simulink model "ZynqBF_2tx_fpga"  (R2018b)
settings: Solver=FixedStepDiscrete  StartTime=0.0  StopTime=10.0  FixedStep=(1/420e3)/128  RelTol=1e-3
undefined symbols (not defined in the file): a, b, c, gs1_i, gs1_q, gs2_i, gs2_q, gs_length
libraries: hdlsllib x65, simulink x41
(part 1 of 4)
settings Model: DataTypeOverride=Off  Creator=jason  LastModifiedBy=meyer
settings DataIOCC: SaveOutput=off  SaveTime=off
settings OptimizationCC: BlockReduction=off  ConditionallyExecuteInputs=off  DefaultParameterBehavior=Inlined
settings DebuggingCC: AlgebraicLoopMsg=error  SingleTaskRateTransMsg=error  ParameterPrecisionLossMsg=none  StrictBusMsg=ErrorOnBusTreatedAsVector
settings HardwareCC: ProdBitPerPointer=32  ProdBitPerSizeT=32  ProdBitPerPtrDiffT=32  ProdLargestAtomicFloat=None  ProdIntDivRoundTo=Undefined  ProdEndianess=Unspecified  ProdWordSize=32  ProdHWDeviceType=ASIC/FPGA->ASIC/FPGA  ProdEqTarget=off
settings SFSimCC: SimUseLocalCustomCode=off
settings RTWCC: RTWUseLocalCustomCode=off
settings CodeAppCC: StateflowObjectComments=on
settings GRTTargetCC: TargetLangStandard=C89/C90 (ANSI)

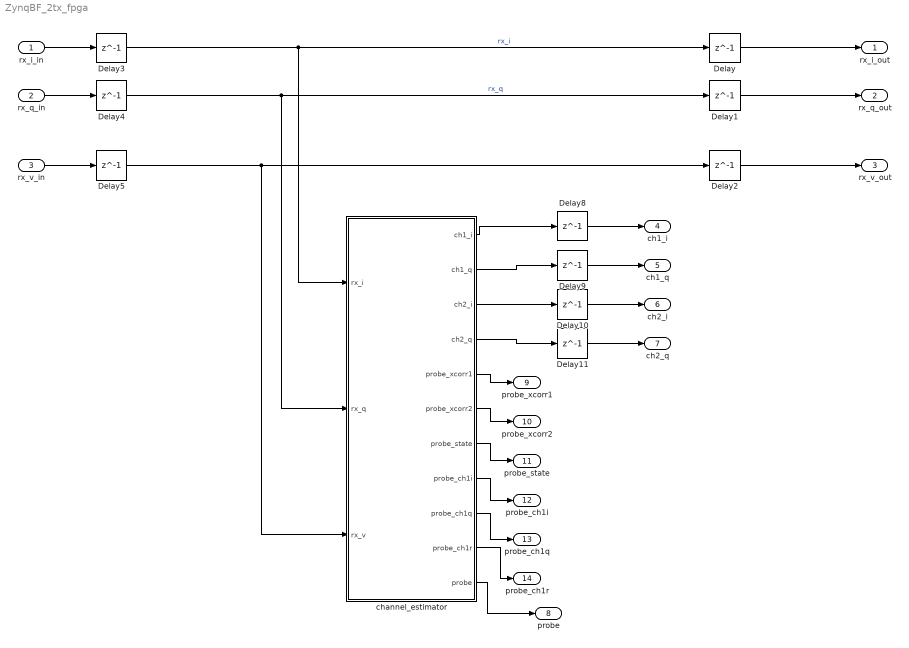
== system ZynqBF_2tx_fpga ==
  rx_i_in : Inport  OutDataTypeStr=fixdt(1,16,15)  SampleTime=1/420e3
  rx_q_in : Inport  Port=2  OutDataTypeStr=fixdt(1,16,15)  SampleTime=1/420e3
  rx_v_in : Inport  Port=3  OutDataTypeStr=boolean  SampleTime=1/420e3
  Delay{,1..5,8..11} (10 alike) : Delay  DelayLength=1
  channel_estimator : Subsystem  TreatAsAtomicUnit=on
  rx_i_out : Outport  OutDataTypeStr=fixdt(1,16,15)  SampleTime=1/420e3
  rx_q_out : Outport  Port=2  OutDataTypeStr=fixdt(1,16,15)  SampleTime=1/420e3
  rx_v_out : Outport  Port=3  OutDataTypeStr=boolean  SampleTime=1/420e3  LockScale=on
  ch1_i : Outport  Port=4  OutDataTypeStr=fixdt(1,16,15)
  ch1_q : Outport  Port=5  OutDataTypeStr=fixdt(1,16,15)
  ch2_i : Outport  Port=6  OutDataTypeStr=fixdt(1,16,15)
  ch2_q : Outport  Port=7  OutDataTypeStr=fixdt(1,16,15)
  probe : Outport  Port=8
  probe_xcorr1 : Outport  Port=9
  probe_xcorr2 : Outport  Port=10
  probe_state : Outport  Port=11
  probe_ch1i : Outport  Port=12
  probe_ch1q : Outport  Port=13
  probe_ch1r : Outport  Port=14
  wires:
  rx_i_in/1 -> Delay3/1
  rx_q_in/1 -> Delay4/1
  rx_v_in/1 -> Delay5/1
  Delay/1 -> rx_i_out/1
  Delay1/1 -> rx_q_out/1
  Delay2/1 -> rx_v_out/1
  channel_estimator/1(ch1_i) -> Delay8/1
  channel_estimator/2(ch1_q) -> Delay9/1
  channel_estimator/3(ch2_i) -> Delay10/1
  channel_estimator/4(ch2_q) -> Delay11/1
  Delay4/1 -> channel_estimator/2(rx_q), Delay1/1  "rx_q"
  Delay5/1 -> channel_estimator/3(rx_v), Delay2/1
  Delay8/1 -> ch1_i/1
  Delay9/1 -> ch1_q/1
  Delay10/1 -> ch2_i/1
  Delay11/1 -> ch2_q/1
  Delay3/1 -> channel_estimator/1(rx_i), Delay/1  "rx_i"
  channel_estimator/5(probe_xcorr1) -> probe_xcorr1/1
  channel_estimator/6(probe_xcorr2) -> probe_xcorr2/1
  channel_estimator/7(probe_state) -> probe_state/1
  channel_estimator/8(probe_ch1i) -> probe_ch1i/1
  channel_estimator/9(probe_ch1q) -> probe_ch1q/1
  channel_estimator/10(probe_ch1r) -> probe_ch1r/1
  channel_estimator/11(probe) -> probe/1

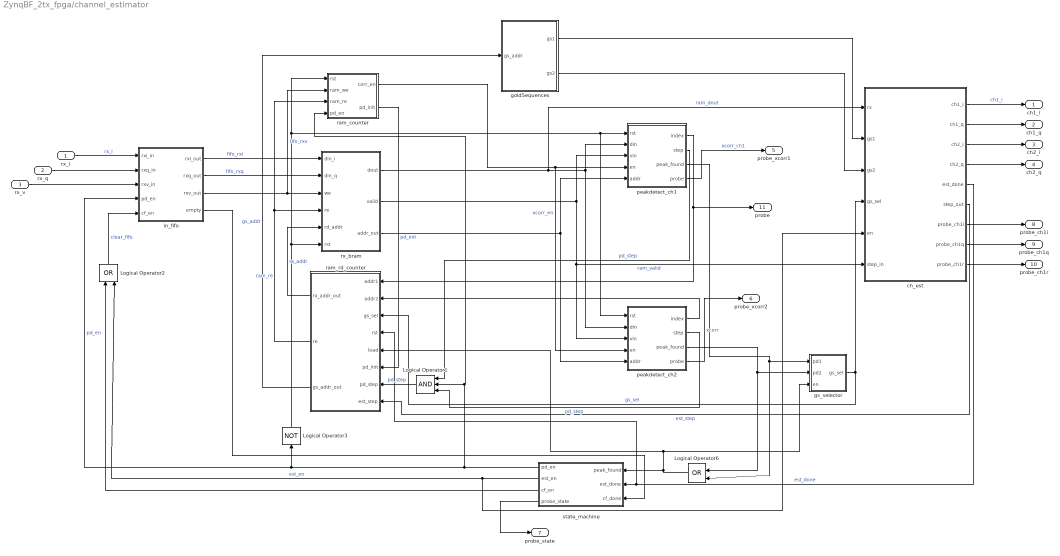
== system ZynqBF_2tx_fpga/channel_estimator ==
  rx_i : Inport
  rx_q : Inport  Port=2
  rx_v : Inport  Port=3
  Logical Operator1 : Logic  Inputs=3  IconShape=distinctive  AllPortsSameDT=off  OutDataTypeStr=boolean
  Logical Operator2 : Logic  Operator=OR  IconShape=distinctive  AllPortsSameDT=off  OutDataTypeStr=boolean
  Logical Operator3 : Logic  Operator=NOT  IconShape=distinctive  AllPortsSameDT=off  OutDataTypeStr=boolean
  Logical Operator6 : Logic  Operator=OR  IconShape=distinctive  AllPortsSameDT=off  OutDataTypeStr=boolean
  ch_est : Subsystem
  goldSequences : Subsystem
  gs_selector : Subsystem
  in_fifo : Subsystem
  peakdetect_ch1 : Subsystem
  peakdetect_ch2 : Subsystem
  ram_counter : Subsystem
  ram_rd_counter : Subsystem
  rx_bram : Subsystem
  state_machine : Subsystem
  ch1_i : Outport
  ch1_q : Outport  Port=2
  ch2_i : Outport  Port=3
  ch2_q : Outport  Port=4
  probe_xcorr1 : Outport  Port=5
  probe_xcorr2 : Outport  Port=6
  probe_state : Outport  Port=7
  probe_ch1i : Outport  Port=8
  probe_ch1q : Outport  Port=9
  probe_ch1r : Outport  Port=10
  probe : Outport  Port=11
  wires:
  in_fifo/3(rxv_out) -> ram_counter/2(ram_we), rx_bram/3(we)  "fifo_rxv"
  peakdetect_ch1/2(step) -> Logical Operator1/1  "pd_step"
  rx_bram/1(dout) -> ch_est/1(rx), peakdetect_ch2/2(din), peakdetect_ch1/2(din)  "ram_dout"
  goldSequences/1(gs1) -> ch_est/2(gs1)
  state_machine/1(pd_en) -> Logical Operator3/1, in_fifo/4(pd_en), ram_counter/4(pd_en), Logical Operator1/2  "pd_en"
  Logical Operator6/1 -> state_machine/1(peak_found), ram_rd_counter/5(load), gs_selector/3(en)
  ch_est/5(est_done) -> ram_rd_counter/4(rst), state_machine/2(est_done)  "est_done"
  goldSequences/2(gs2) -> ch_est/3(gs2)
  peakdetect_ch2/3(peak_found) -> Logical Operator6/1, gs_selector/2(pd2)
  peakdetect_ch1/3(peak_found) -> Logical Operator6/2, gs_selector/1(pd1)
  gs_selector/1(gs_sel) -> ch_est/4(gs_sel), ram_rd_counter/3(gs_sel)  "gs_sel"
  ch_est/1(ch1_i) -> ch1_i/1  "ch1_i"
  ch_est/2(ch1_q) -> ch1_q/1
  ch_est/3(ch2_i) -> ch2_i/1
  ch_est/4(ch2_q) -> ch2_q/1
  rx_bram/2(valid) -> peakdetect_ch2/3(vin), ch_est/6(step_in), peakdetect_ch1/3(vin)  "ram_valid"
  ram_rd_counter/1(rx_addr_out) -> rx_bram/5(rd_addr)  "rx_addr"
  ram_rd_counter/2(re) -> ram_counter/3(ram_re), rx_bram/4(re)  "ram_re"
  state_machine/2(est_en) -> ch_est/5(en), Logical Operator2/2  "est_en"
  rx_bram/3(addr_out) -> peakdetect_ch2/5(addr), peakdetect_ch1/5(addr)
  ram_rd_counter/3(gs_addr_out) -> goldSequences/1(gs_addr)  "gs_addr"
  ch_est/6(step_out) -> ram_rd_counter/8(est_step)  "est_step"
  peakdetect_ch2/2(step) -> Logical Operator1/3  "pd_step"
  peakdetect_ch1/1(index) -> probe/1, ram_rd_counter/1(addr1)
  peakdetect_ch2/1(index) -> ram_rd_counter/2(addr2)
  peakdetect_ch2/4(probe) -> probe_xcorr2/1  "xcorr"
  state_machine/3(cf_en) -> Logical Operator2/1
  peakdetect_ch1/4(probe) -> probe_xcorr1/1  "xcorr_ch1"
  ram_counter/1(corr_en) -> peakdetect_ch2/4(en), peakdetect_ch1/4(en)  "xcorr_en"
  in_fifo/1(rxi_out) -> rx_bram/1(din_i)  "fifo_rxi"
  in_fifo/2(rxq_out) -> rx_bram/2(din_q)  "fifo_rxq"
  rx_i/1 -> in_fifo/1(rxi_in)  "rx_i"
  rx_q/1 -> in_fifo/2(rxq_in)
  rx_v/1 -> in_fifo/3(rxv_in)
  in_fifo/4(empty) -> state_machine/3(cf_done)
  Logical Operator2/1 -> in_fifo/5(cf_en)  "clear_fifo"
  ch_est/7(probe_ch1i) -> probe_ch1i/1
  ch_est/8(probe_ch1q) -> probe_ch1q/1
  ch_est/9(probe_ch1r) -> probe_ch1r/1
  state_machine/4(probe_state) -> probe_state/1
  Logical Operator3/1 -> ram_counter/1(rst), peakdetect_ch2/1(rst), peakdetect_ch1/1(rst), rx_bram/6(rst)
  ram_counter/2(pd_init) -> ram_rd_counter/6(pd_init)  "pd_init"
  Logical Operator1/1 -> ram_rd_counter/7(pd_step)  "pd_step"

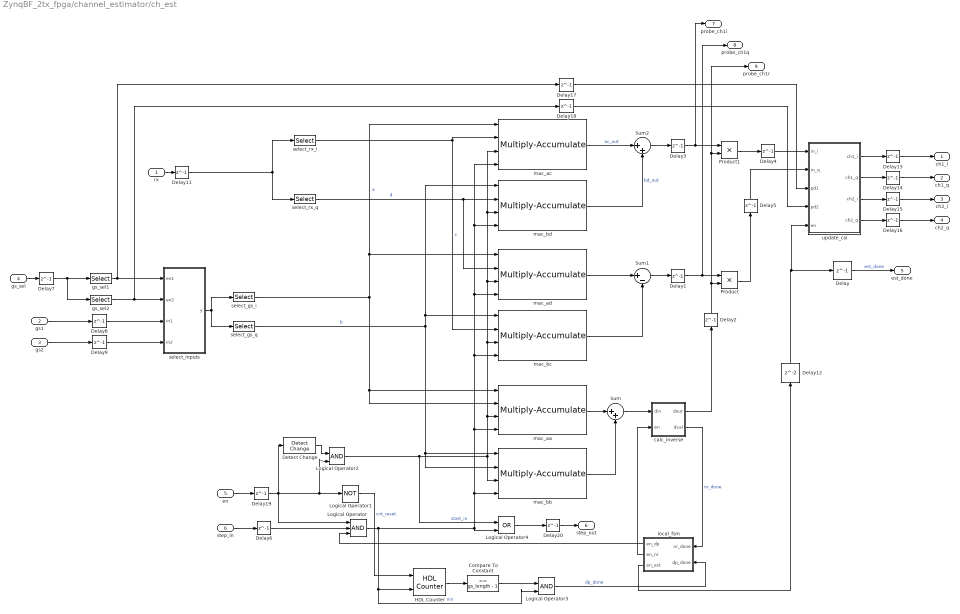
== system ZynqBF_2tx_fpga/channel_estimator/ch_est ==
  rx : Inport
  gs1 : Inport  Port=2
  gs2 : Inport  Port=3
  gs_sel : Inport  Port=4
  en : Inport  Port=5
  step_in : Inport  Port=6
  Compare To Constant : simulink/Logic and Bit Operations/Compare To Constant  relop===  const=gs_length - 1  OutDataTypeStr=boolean
  Delay{,1..9,11,13..20} (19 alike) : Delay  DelayLength=1
  Delay12 : Delay
  Detect Change : simulink/Logic and Bit Operations/Detect Change  vinit=0  OutDataTypeStr=boolean
  HDL Counter : hdlsllib/Sources/HDL Counter  CountType=Count limited  CountInit=0  CountStep=1  CountMax=gs_length-1  CountFromType=Initial value  CountFrom=0  CountResetPort=on  CountLoadPort=off  CountEnbPort=on  CountDirPort=off  CountDataType=Unsigned  CountWordLen=16  CountFracLen=0  CountSampTime=-1
      settings: SourceProductBaseCode=HD
  Logical Operator : Logic  Inputs=3  IconShape=distinctive  AllPortsSameDT=off  OutDataTypeStr=boolean
  Logical Operator1 : Logic  Operator=NOT  IconShape=distinctive  AllPortsSameDT=off  OutDataTypeStr=boolean
  Logical Operator2 : Logic  IconShape=distinctive  AllPortsSameDT=off  OutDataTypeStr=boolean
  Logical Operator3 : Logic  IconShape=distinctive  AllPortsSameDT=off  OutDataTypeStr=boolean
  Logical Operator4 : Logic  Operator=OR  IconShape=distinctive  AllPortsSameDT=off  OutDataTypeStr=boolean
  Product : Product  OutDataTypeStr=fixdt(1,16,15)
  Product1 : Product  OutDataTypeStr=fixdt(1,16,15)
  Sum : Sum  Inputs=|++  OutDataTypeStr=fixdt(1,32,16)
  Sum1 : Sum  Inputs=|+-  OutDataTypeStr=fixdt(1,32,16)
  Sum2 : Sum  Inputs=|++  OutDataTypeStr=fixdt(1,32,16)
  calc_inverse : Subsystem
  gs_sel1 : Selector  IndexMode=Zero-based  InputPortWidth=2  IndexOptions=Index vector (dialog)  Indices=[0]  OutputSizes=1
  gs_sel2 : Selector  IndexMode=Zero-based  InputPortWidth=2  IndexOptions=Index vector (dialog)  Indices=[1]  OutputSizes=1
  local_fsm : Subsystem
  mac_aa : hdlsllib/HDL Operations/Multiply-Accumulate  opMode=Streaming - using Start and End ports  initValueSetting=Dialog  initValue=0  initValueSetting2=Dialog  initValue2=0  initValueSetting3=Dialog  initValue3=0  num_samples=2048  RndMeth2=Floor  RndMeth3=Floor  datatype2=fixdt(1,32,16)  datatype3=Inherit: Inherit via back propagation  validOut=off  endInandOut=off  startOut=off  countOut=off  dim=-1  DoSatur=off  parallel=off
      settings: SourceProductName=HDL Coder  SourceProductBaseCode=HD
  mac_ac : hdlsllib/HDL Operations/Multiply-Accumulate  opMode=Streaming - using Start and End ports  initValueSetting=Dialog  initValue=0  initValueSetting2=Dialog  initValue2=0  initValueSetting3=Dialog  initValue3=0  num_samples=2048  RndMeth2=Floor  RndMeth3=Floor  datatype2=fixdt(1,32,16)  datatype3=Inherit: Inherit via back propagation  validOut=off  endInandOut=off  startOut=off  countOut=off  dim=-1  DoSatur=off  parallel=off
      settings: SourceProductName=HDL Coder  SourceProductBaseCode=HD
  mac_ad : hdlsllib/HDL Operations/Multiply-Accumulate  opMode=Streaming - using Start and End ports  initValueSetting=Dialog  initValue=0  initValueSetting2=Dialog  initValue2=0  initValueSetting3=Dialog  initValue3=0  num_samples=2048  RndMeth2=Floor  RndMeth3=Floor  datatype2=fixdt(1,32,16)  datatype3=Inherit: Inherit via back propagation  validOut=off  endInandOut=off  startOut=off  countOut=off  dim=-1  DoSatur=off  parallel=off
      settings: SourceProductName=HDL Coder  SourceProductBaseCode=HD
  mac_bb : hdlsllib/HDL Operations/Multiply-Accumulate  opMode=Streaming - using Start and End ports  initValueSetting=Dialog  initValue=0  initValueSetting2=Dialog  initValue2=0  initValueSetting3=Dialog  initValue3=0  num_samples=2048  RndMeth2=Floor  RndMeth3=Floor  datatype2=fixdt(1,32,16)  datatype3=Inherit: Inherit via back propagation  validOut=off  endInandOut=off  startOut=off  countOut=off  dim=-1  DoSatur=off  parallel=off
      settings: SourceProductName=HDL Coder  SourceProductBaseCode=HD
  mac_bc : hdlsllib/HDL Operations/Multiply-Accumulate  opMode=Streaming - using Start and End ports  initValueSetting=Dialog  initValue=0  initValueSetting2=Dialog  initValue2=0  initValueSetting3=Dialog  initValue3=0  num_samples=2048  RndMeth2=Floor  RndMeth3=Floor  datatype2=fixdt(1,32,16)  datatype3=Inherit: Inherit via back propagation  validOut=off  endInandOut=off  startOut=off  countOut=off  dim=-1  DoSatur=off  parallel=off
      settings: SourceProductName=HDL Coder  SourceProductBaseCode=HD
  mac_bd : hdlsllib/HDL Operations/Multiply-Accumulate  opMode=Streaming - using Start and End ports  initValueSetting=Dialog  initValue=0  initValueSetting2=Dialog  initValue2=0  initValueSetting3=Dialog  initValue3=0  num_samples=2048  RndMeth2=Floor  RndMeth3=Floor  datatype2=fixdt(1,32,16)  datatype3=Inherit: Inherit via back propagation  validOut=off  endInandOut=off  startOut=off  countOut=off  dim=-1  DoSatur=off  parallel=off
      settings: SourceProductName=HDL Coder  SourceProductBaseCode=HD
  select_gs_i : Selector  IndexMode=Zero-based  InputPortWidth=2  IndexOptions=Index vector (dialog)  Indices=[0]  OutputSizes=1
  select_gs_q : Selector  IndexMode=Zero-based  InputPortWidth=2  IndexOptions=Index vector (dialog)  Indices=[1]  OutputSizes=1
  select_inputs : MATLAB Function  TreatAsAtomicUnit=on
  select_rx_i : Selector  IndexMode=Zero-based  InputPortWidth=2  IndexOptions=Index vector (dialog)  Indices=[0]  OutputSizes=1
  select_rx_q : Selector  IndexMode=Zero-based  InputPortWidth=2  IndexOptions=Index vector (dialog)  Indices=[1]  OutputSizes=1
  update_csi : Subsystem
  ch1_i : Outport
  ch1_q : Outport  Port=2
  ch2_i : Outport  Port=3
  ch2_q : Outport  Port=4
  est_done : Outport  Port=5
  step_out : Outport  Port=6
  probe_ch1i : Outport  Port=7
  probe_ch1q : Outport  Port=8
  probe_ch1r : Outport  Port=9
  wires:
  gs_sel/1 -> Delay7/1
  select_rx_i/1 -> mac_bc/2, mac_ac/2  "c"
  select_rx_q/1 -> mac_ad/2, mac_bd/2  "d"
  Logical Operator/1 -> Logical Operator4/2, mac_ac/4, mac_bd/4, mac_ad/4, mac_bc/4, mac_aa/4, mac_bb/4, Logical Operator3/2, HDL Counter/2  "vin"
  gs1/1 -> Delay8/1
  gs2/1 -> Delay9/1
  select_inputs/1(y) -> select_gs_q/1, select_gs_i/1
  mac_ad/1 -> Sum1/1
  mac_bc/1 -> Sum1/2
  mac_ac/1 -> Sum2/1  "ac_out"
  mac_bd/1 -> Sum2/2  "bd_out"
  step_in/1 -> Delay6/1
  local_fsm/1(en_dp) -> Logical Operator/3
  Sum/1 -> calc_inverse/1(din)
  calc_inverse/2(dval) -> local_fsm/1(nr_done)  "nr_done"
  local_fsm/2(en_nr) -> calc_inverse/2(en)
  calc_inverse/1(dout) -> Delay2/1
  Sum1/1 -> Delay1/1
  Sum2/1 -> Delay3/1
  local_fsm/3(en_est) -> Delay12/1
  Product1/1 -> Delay4/1
  Product/1 -> Delay5/1
  update_csi/1(ch1_i) -> Delay13/1
  update_csi/2(ch1_q) -> Delay14/1
  update_csi/3(ch2_i) -> Delay15/1
  update_csi/4(ch2_q) -> Delay16/1
  Delay/1 -> est_done/1  "est_done"
  rx/1 -> Delay11/1
  Delay11/1 -> select_rx_i/1, select_rx_q/1
  Delay2/1 -> probe_ch1r/1, Product1/2, Product/2
  Delay1/1 -> probe_ch1q/1, Product/1
  Delay3/1 -> probe_ch1i/1, Product1/1
  Delay4/1 -> update_csi/1(in_i)
  Delay5/1 -> update_csi/2(in_q)
  Delay6/1 -> Logical Operator/2
  Delay8/1 -> select_inputs/3(in1)
  Delay9/1 -> select_inputs/4(in2)
  Delay12/1 -> Delay/1, update_csi/5(en)
  Delay13/1 -> ch1_i/1
  Delay14/1 -> ch1_q/1
  Delay15/1 -> ch2_i/1
  Delay16/1 -> ch2_q/1
  Delay7/1 -> gs_sel2/1, gs_sel1/1
  gs_sel2/1 -> Delay18/1, select_inputs/2(en2)
  gs_sel1/1 -> Delay17/1, select_inputs/1(en1)
  Delay17/1 -> update_csi/3(pd1)
  Delay18/1 -> update_csi/4(pd2)
  select_gs_i/1 -> mac_aa/1, mac_aa/2, mac_ac/1, mac_ad/1  "a"
  select_gs_q/1 -> mac_bb/2, mac_bb/1, mac_bd/1, mac_bc/1  "b"
  en/1 -> Delay19/1
  Logical Operator1/1 -> HDL Counter/1  "cnt_reset"
  Delay19/1 -> Logical Operator/1, Detect Change/1, Logical Operator2/2, Logical Operator1/1
  Detect Change/1 -> Logical Operator2/1
  Logical Operator2/1 -> Logical Operator4/1, mac_bb/3, mac_aa/3, mac_bc/3, mac_ad/3, mac_bd/3, mac_ac/3  "start_in"
  HDL Counter/1 -> Compare To Constant/1
  mac_aa/1 -> Sum/1
  mac_bb/1 -> Sum/2
  Delay20/1 -> step_out/1
  Compare To Constant/1 -> Logical Operator3/1
  Logical Operator3/1 -> local_fsm/2(dp_done)  "dp_done"
  Logical Operator4/1 -> Delay20/1

== system ZynqBF_2tx_fpga/channel_estimator/goldSequences ==
  gs_addr : Inport
  Delay{2..6,8,11} (7 alike) : Delay  DelayLength=1
  Vector Concatenate1 : Concatenate
  Vector Concatenate2 : Concatenate
  gs1_i : Lookup_n-D  NumberOfTableDimensions=1  LookupTableObject=''  BreakpointsForDimension1=[0:(gs_length-1)]  BreakpointsForDimension1FirstPoint=10  BreakpointsForDimension2FirstPoint=10  BreakpointsForDimension1Spacing=12  BreakpointsForDimension2Spacing=12  IndexSearchMethod=Evenly spaced points  Table=gs1_i  InterpMethod=Flat  DiagnosticForOutOfRangeInput=Error  InternalRulePriority=Speed  OutDataTypeStr=fixdt(1,16,15)  RndMeth=Simplest  InputSameDT=on
  gs1_q : Lookup_n-D  NumberOfTableDimensions=1  LookupTableObject=''  BreakpointsForDimension1=[0:(gs_length-1)]  BreakpointsForDimension1FirstPoint=10  BreakpointsForDimension2FirstPoint=10  BreakpointsForDimension1Spacing=12  BreakpointsForDimension2Spacing=12  IndexSearchMethod=Evenly spaced points  Table=gs1_q  InterpMethod=Flat  DiagnosticForOutOfRangeInput=Error  InternalRulePriority=Speed  OutDataTypeStr=fixdt(1,16,15)  RndMeth=Simplest  InputSameDT=on
  gs2_i : Lookup_n-D  NumberOfTableDimensions=1  LookupTableObject=''  BreakpointsForDimension1=[0:(gs_length-1)]  BreakpointsForDimension1FirstPoint=10  BreakpointsForDimension2FirstPoint=10  BreakpointsForDimension1Spacing=12  BreakpointsForDimension2Spacing=12  IndexSearchMethod=Evenly spaced points  Table=gs2_i  InterpMethod=Flat  DiagnosticForOutOfRangeInput=Error  InternalRulePriority=Speed  OutDataTypeStr=fixdt(1,16,15)  RndMeth=Simplest  InputSameDT=on
  gs2_q : Lookup_n-D  NumberOfTableDimensions=1  LookupTableObject=''  BreakpointsForDimension1=[0:(gs_length-1)]  BreakpointsForDimension1FirstPoint=10  BreakpointsForDimension2FirstPoint=10  BreakpointsForDimension1Spacing=12  BreakpointsForDimension2Spacing=12  IndexSearchMethod=Evenly spaced points  Table=gs2_q  InterpMethod=Flat  DiagnosticForOutOfRangeInput=Error  InternalRulePriority=Speed  OutDataTypeStr=fixdt(1,16,15)  RndMeth=Simplest  InputSameDT=on
  gs1 : Outport
  gs2 : Outport  Port=2
  wires:
  gs2_q/1 -> Delay3/1
  gs2_i/1 -> Delay2/1
  Delay2/1 -> Vector Concatenate1/1
  Delay3/1 -> Vector Concatenate1/2
  gs_addr/1 -> Delay4/1
  gs1_i/1 -> Delay5/1
  Delay5/1 -> Vector Concatenate2/1
  Delay6/1 -> gs1/1
  Delay4/1 -> gs1_q/1, gs2_q/1, gs2_i/1, gs1_i/1
  gs1_q/1 -> Delay8/1
  Delay8/1 -> Vector Concatenate2/2
  Vector Concatenate2/1 -> Delay6/1
  Delay11/1 -> gs2/1
  Vector Concatenate1/1 -> Delay11/1

== system ZynqBF_2tx_fpga/channel_estimator/gs_selector ==
  pd1 : Inport
  pd2 : Inport  Port=2
  en : Inport  Port=3
  Delay{1..5} (5 alike) : Delay  DelayLength=1
  Switch1 : Switch  Criteria=u2 ~= 0
  Vector Concatenate : Concatenate
  gs_sel : Outport
  wires:
  pd2/1 -> Delay2/1
  en/1 -> Delay4/1
  pd1/1 -> Delay1/1
  Delay2/1 -> Vector Concatenate/2
  Delay1/1 -> Vector Concatenate/1
  Delay3/1 -> gs_sel/1
  Switch1/1 -> Delay3/1, Delay5/1
  Delay4/1 -> Switch1/2
  Vector Concatenate/1 -> Switch1/1
  Delay5/1 -> Switch1/3

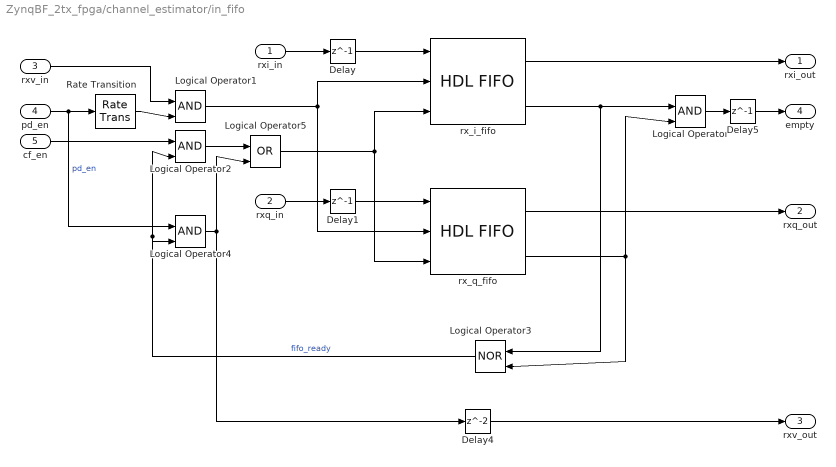
== system ZynqBF_2tx_fpga/channel_estimator/in_fifo ==
  rxi_in : Inport
  rxq_in : Inport  Port=2
  rxv_in : Inport  Port=3
  pd_en : Inport  Port=4
  cf_en : Inport  Port=5
  Delay : Delay  DelayLength=1
  Delay1 : Delay  DelayLength=1
  Delay4 : Delay
  Delay5 : Delay  DelayLength=1
  Logical Operator{,1..2,4} (4 alike) : Logic  IconShape=distinctive  AllPortsSameDT=off  OutDataTypeStr=boolean
  Logical Operator3 : Logic  Operator=NOR  IconShape=distinctive  AllPortsSameDT=off  OutDataTypeStr=boolean
  Logical Operator5 : Logic  Operator=OR  IconShape=distinctive  AllPortsSameDT=off  OutDataTypeStr=boolean
  Rate Transition : RateTransition
  rx_i_fifo : hdlsllib/HDL RAMs/HDL FIFO  fifo_size=8912  ratio=1/128  push_msg=Warning  pop_msg=Warning  show_empty=on  show_full=off  show_num=off
      settings: SourceProductName=HDL Coder  SourceProductBaseCode=HD
  rx_q_fifo : hdlsllib/HDL RAMs/HDL FIFO  fifo_size=8912  ratio=1/128  push_msg=Warning  pop_msg=Warning  show_empty=on  show_full=off  show_num=off
      settings: SourceProductName=HDL Coder  SourceProductBaseCode=HD
  rxi_out : Outport
  rxq_out : Outport  Port=2
  rxv_out : Outport  Port=3
  empty : Outport  Port=4
  wires:
  Logical Operator5/1 -> rx_i_fifo/3, rx_q_fifo/3
  rxi_in/1 -> Delay/1
  rx_q_fifo/2 -> Logical Operator3/2, Logical Operator/2
  rx_i_fifo/1 -> rxi_out/1
  Logical Operator1/1 -> rx_i_fifo/2, rx_q_fifo/2
  rxq_in/1 -> Delay1/1
  rx_q_fifo/1 -> rxq_out/1
  Logical Operator/1 -> Delay5/1
  rx_i_fifo/2 -> Logical Operator3/1, Logical Operator/1
  Delay/1 -> rx_i_fifo/1
  Delay1/1 -> rx_q_fifo/1
  rxv_in/1 -> Logical Operator1/1
  Logical Operator3/1 -> Logical Operator2/2, Logical Operator4/2  "fifo_ready"
  Delay5/1 -> empty/1
  pd_en/1 -> Logical Operator4/1, Rate Transition/1  "pd_en"
  cf_en/1 -> Logical Operator2/1
  Logical Operator4/1 -> Logical Operator5/2, Delay4/1
  Logical Operator2/1 -> Logical Operator5/1
  Delay4/1 -> rxv_out/1
  Rate Transition/1 -> Logical Operator1/2

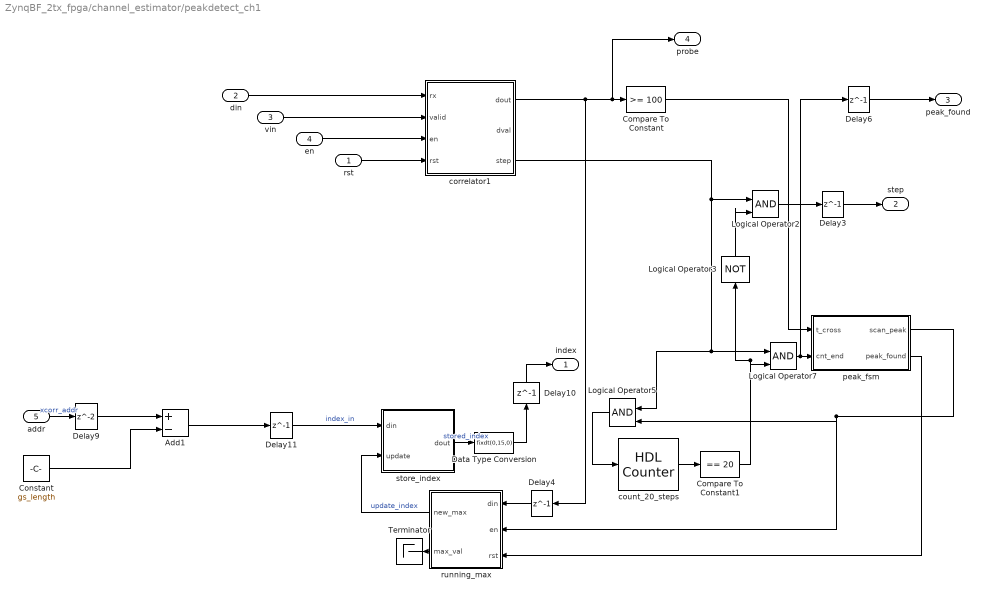
== system ZynqBF_2tx_fpga/channel_estimator/peakdetect_ch1 ==
  rst : Inport
  din : Inport  Port=2
  vin : Inport  Port=3
  en : Inport  Port=4
  addr : Inport  Port=5
  Add1 : Sum  Inputs=+-  OutDataTypeStr=int16
  Compare To Constant : simulink/Logic and Bit Operations/Compare To Constant  relop=>=  const=100  OutDataTypeStr=boolean
  Compare To Constant1 : simulink/Logic and Bit Operations/Compare To Constant  relop===  const=20  OutDataTypeStr=boolean
  Constant : Constant  Value=gs_length  OutDataTypeStr=uint16  SampleTime=-1
  Data Type Conversion : DataTypeConversion  OutDataTypeStr=fixdt(0,15,0)
  Delay{3..4,6,10..11} (5 alike) : Delay  DelayLength=1
  Delay9 : Delay
  Logical Operator2 : Logic  IconShape=distinctive  AllPortsSameDT=off  OutDataTypeStr=boolean
  Logical Operator3 : Logic  Operator=NOT  IconShape=distinctive  AllPortsSameDT=off  OutDataTypeStr=boolean
  Logical Operator5 : Logic  IconShape=distinctive  AllPortsSameDT=off  OutDataTypeStr=boolean
  Logical Operator7 : Logic  IconShape=distinctive  AllPortsSameDT=off  OutDataTypeStr=boolean
  Terminator : Terminator
  correlator1 : Subsystem
  count_20_steps : hdlsllib/Sources/HDL Counter  CountType=Count limited  CountInit=0  CountStep=1  CountMax=20  CountFromType=Initial value  CountFrom=0  CountResetPort=off  CountLoadPort=off  CountEnbPort=on  CountDirPort=off  CountDataType=Unsigned  CountWordLen=8  CountFracLen=0  CountSampTime=1
      settings: SourceProductBaseCode=HD
  peak_fsm : Subsystem
  running_max : Subsystem
  store_index : Subsystem
  index : Outport
  step : Outport  Port=2
  peak_found : Outport  Port=3
  probe : Outport  Port=4
  wires:
  rst/1 -> correlator1/4(rst)
  en/1 -> correlator1/3(en)
  vin/1 -> correlator1/2(valid)
  din/1 -> correlator1/1(rx)
  Compare To Constant1/1 -> Logical Operator3/1, Logical Operator7/2
  Delay6/1 -> peak_found/1
  Logical Operator7/1 -> Delay6/1, peak_fsm/2(cnt_end)
  count_20_steps/1 -> Compare To Constant1/1
  Logical Operator5/1 -> count_20_steps/1
  peak_fsm/1(scan_peak) -> running_max/2(en), Logical Operator5/2
  Compare To Constant/1 -> peak_fsm/1(t_cross)
  Data Type Conversion/1 -> Delay10/1
  Add1/1 -> Delay11/1
  Delay3/1 -> step/1
  Delay10/1 -> index/1
  Delay11/1 -> store_index/1(din)  "index_in"
  correlator1/3(step) -> Logical Operator2/1, Logical Operator5/1, Logical Operator7/1
  Logical Operator3/1 -> Logical Operator2/2
  Delay9/1 -> Add1/1
  Logical Operator2/1 -> Delay3/1
  peak_fsm/2(peak_found) -> running_max/3(rst)
  running_max/2(max_val) -> Terminator/1
  correlator1/1(dout) -> probe/1, Compare To Constant/1, Delay4/1
  Delay4/1 -> running_max/1(din)
  running_max/1(new_max) -> store_index/2(update)  "update_index"
  Constant/1 -> Add1/2
  addr/1 -> Delay9/1  "xcorr_addr"
  store_index/1(dout) -> Data Type Conversion/1  "stored_index"

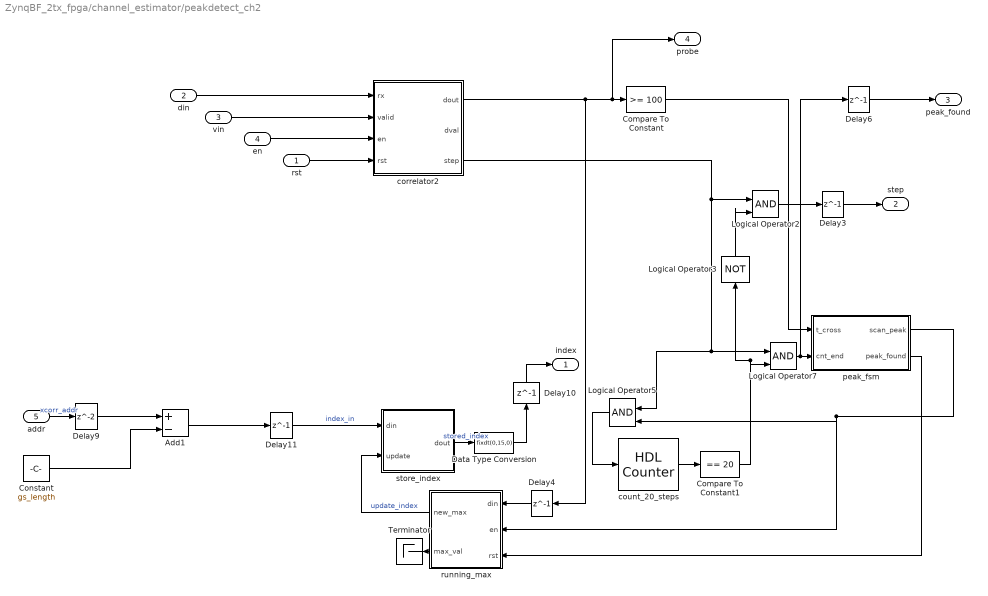
== system ZynqBF_2tx_fpga/channel_estimator/peakdetect_ch2 ==
  rst : Inport
  din : Inport  Port=2
  vin : Inport  Port=3
  en : Inport  Port=4
  addr : Inport  Port=5
  Add1 : Sum  Inputs=+-  OutDataTypeStr=int16
  Compare To Constant : simulink/Logic and Bit Operations/Compare To Constant  relop=>=  const=100  OutDataTypeStr=boolean
  Compare To Constant1 : simulink/Logic and Bit Operations/Compare To Constant  relop===  const=20  OutDataTypeStr=boolean
  Constant : Constant  Value=gs_length  OutDataTypeStr=uint16  SampleTime=-1
  Data Type Conversion : DataTypeConversion  OutDataTypeStr=fixdt(0,15,0)
  Delay{3..4,6,10..11} (5 alike) : Delay  DelayLength=1
  Delay9 : Delay
  Logical Operator2 : Logic  IconShape=distinctive  AllPortsSameDT=off  OutDataTypeStr=boolean
  Logical Operator3 : Logic  Operator=NOT  IconShape=distinctive  AllPortsSameDT=off  OutDataTypeStr=boolean
  Logical Operator5 : Logic  IconShape=distinctive  AllPortsSameDT=off  OutDataTypeStr=boolean
  Logical Operator7 : Logic  IconShape=distinctive  AllPortsSameDT=off  OutDataTypeStr=boolean
  Terminator : Terminator
  correlator2 : Subsystem
  count_20_steps : hdlsllib/Sources/HDL Counter  CountType=Count limited  CountInit=0  CountStep=1  CountMax=20  CountFromType=Initial value  CountFrom=0  CountResetPort=off  CountLoadPort=off  CountEnbPort=on  CountDirPort=off  CountDataType=Unsigned  CountWordLen=8  CountFracLen=0  CountSampTime=1
      settings: SourceProductBaseCode=HD
  peak_fsm : Subsystem
  running_max : Subsystem
  store_index : Subsystem
  index : Outport
  step : Outport  Port=2
  peak_found : Outport  Port=3
  probe : Outport  Port=4
  wires:
  store_index/1(dout) -> Data Type Conversion/1  "stored_index"
  addr/1 -> Delay9/1  "xcorr_addr"
  Constant/1 -> Add1/2
  running_max/1(new_max) -> store_index/2(update)  "update_index"
  Delay4/1 -> running_max/1(din)
  correlator2/1(dout) -> Delay4/1, Compare To Constant/1, probe/1
  running_max/2(max_val) -> Terminator/1
  peak_fsm/2(peak_found) -> running_max/3(rst)
  Logical Operator2/1 -> Delay3/1
  Delay9/1 -> Add1/1
  Logical Operator3/1 -> Logical Operator2/2
  correlator2/3(step) -> Logical Operator7/1, Logical Operator5/1, Logical Operator2/1
  Delay11/1 -> store_index/1(din)  "index_in"
  Delay10/1 -> index/1
  Delay3/1 -> step/1
  Add1/1 -> Delay11/1
  Data Type Conversion/1 -> Delay10/1
  Compare To Constant/1 -> peak_fsm/1(t_cross)
  peak_fsm/1(scan_peak) -> Logical Operator5/2, running_max/2(en)
  Logical Operator5/1 -> count_20_steps/1
  count_20_steps/1 -> Compare To Constant1/1
  Logical Operator7/1 -> peak_fsm/2(cnt_end), Delay6/1
  Delay6/1 -> peak_found/1
  Compare To Constant1/1 -> Logical Operator7/2, Logical Operator3/1
  din/1 -> correlator2/1(rx)
  vin/1 -> correlator2/2(valid)
  en/1 -> correlator2/3(en)
  rst/1 -> correlator2/4(rst)

== system ZynqBF_2tx_fpga/channel_estimator/ram_counter ==
  rst : Inport
  ram_we : Inport  Port=2
  ram_re : Inport  Port=3
  pd_en : Inport  Port=4
  Compare To Constant : simulink/Logic and Bit Operations/Compare To Constant  relop=>  const=0  OutDataTypeStr=boolean
  Compare To Constant1 : simulink/Logic and Bit Operations/Compare To Constant  relop===  const=0  OutDataTypeStr=boolean
  Delay{1,4..7} (5 alike) : Delay  DelayLength=1
  Delay2 : Delay  DelayLength=4
  Delay3 : Delay  DelayLength=4
  HDL Counter : hdlsllib/Sources/HDL Counter  CountType=Free running  CountInit=0  CountStep=1  CountMax=25  CountFromType=Initial value  CountFrom=0  CountResetPort=on  CountLoadPort=off  CountEnbPort=on  CountDirPort=on  CountDataType=Unsigned  CountWordLen=16  CountFracLen=0  CountSampTime=1
      settings: SourceProductBaseCode=HD
  HDL Counter1 : hdlsllib/Sources/HDL Counter  CountType=Count limited  CountInit=0  CountStep=1  CountMax=1  CountFromType=Initial value  CountFrom=0  CountResetPort=on  CountLoadPort=off  CountEnbPort=on  CountDirPort=off  CountDataType=Unsigned  CountWordLen=8  CountFracLen=0  CountSampTime=1
      settings: SourceProductBaseCode=HD
  Logical Operator : Logic  Operator=XOR  IconShape=distinctive  AllPortsSameDT=off  OutDataTypeStr=boolean
  Logical Operator1 : Logic  IconShape=distinctive  AllPortsSameDT=off  OutDataTypeStr=boolean
  Logical Operator2 : Logic  IconShape=distinctive  AllPortsSameDT=off  OutDataTypeStr=boolean
  corr_en : Outport
  pd_init : Outport  Port=2
  wires:
  rst/1 -> Delay4/1
  HDL Counter/1 -> Compare To Constant/1  "ram_counter"
  Compare To Constant/1 -> Delay6/1
  ram_we/1 -> Delay1/1
  Delay4/1 -> HDL Counter1/1, HDL Counter/1
  Delay1/1 -> Logical Operator2/1, Logical Operator/2, HDL Counter/3
  ram_re/1 -> Delay2/1
  Logical Operator/1 -> HDL Counter/2
  Delay2/1 -> Logical Operator1/2
  pd_en/1 -> Delay3/1
  Delay3/1 -> Logical Operator1/1
  Logical Operator1/1 -> Delay5/1
  Delay5/1 -> Logical Operator/1
  Delay6/1 -> corr_en/1
  HDL Counter1/1 -> Compare To Constant1/1  "pd_init_count"
  Compare To Constant1/1 -> Logical Operator2/2
  Logical Operator2/1 -> Delay7/1, HDL Counter1/2
  Delay7/1 -> pd_init/1

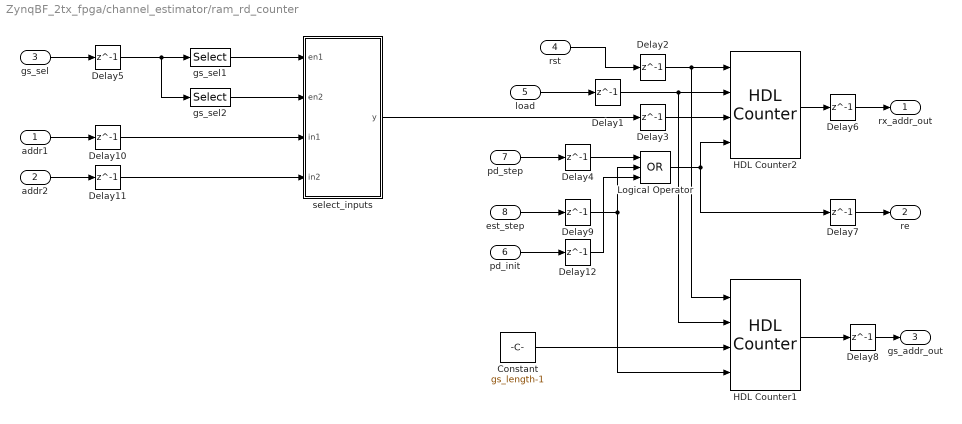
== system ZynqBF_2tx_fpga/channel_estimator/ram_rd_counter ==
  addr1 : Inport
  addr2 : Inport  Port=2
  gs_sel : Inport  Port=3
  rst : Inport  Port=4
  load : Inport  Port=5
  pd_init : Inport  Port=6
  pd_step : Inport  Port=7
  est_step : Inport  Port=8
  Constant : Constant  Value=gs_length-1  OutDataTypeStr=Inherit: Inherit via back propagation  SampleTime=-1
  Delay{1..5,7,9..12} (10 alike) : Delay  DelayLength=1
  Delay6 : Delay  DelayLength=1  InitialCondition=0
  Delay8 : Delay  DelayLength=1  InitialCondition=0
  HDL Counter1 : hdlsllib/Sources/HDL Counter  CountType=Count limited  CountInit=0  CountStep=1  CountMax=gs_length-1  CountFromType=Initial value  CountFrom=0  CountResetPort=on  CountLoadPort=on  CountEnbPort=on  CountDirPort=off  CountDataType=Unsigned  CountWordLen=log(gs_length)/log(2)  CountFracLen=0  CountSampTime=1
      settings: SourceProductBaseCode=HD
  HDL Counter2 : hdlsllib/Sources/HDL Counter  CountType=Count limited  CountInit=0  CountStep=1  CountMax=32767  CountFromType=Initial value  CountFrom=0  CountResetPort=on  CountLoadPort=on  CountEnbPort=on  CountDirPort=off  CountDataType=Unsigned  CountWordLen=15  CountFracLen=0  CountSampTime=1
      settings: SourceProductBaseCode=HD
  Logical Operator : Logic  Operator=OR  Inputs=3  IconShape=distinctive  AllPortsSameDT=off  OutDataTypeStr=boolean
  gs_sel1 : Selector  IndexMode=Zero-based  InputPortWidth=2  IndexOptions=Index vector (dialog)  Indices=[0]  OutputSizes=1
  gs_sel2 : Selector  IndexMode=Zero-based  InputPortWidth=2  IndexOptions=Index vector (dialog)  Indices=[1]  OutputSizes=1
  select_inputs : MATLAB Function  TreatAsAtomicUnit=on
  rx_addr_out : Outport
  re : Outport  Port=2
  gs_addr_out : Outport  Port=3
  wires:
  rst/1 -> Delay2/1
  load/1 -> Delay1/1
  Logical Operator/1 -> HDL Counter2/4, Delay7/1
  select_inputs/1(y) -> Delay3/1
  HDL Counter2/1 -> Delay6/1
  pd_step/1 -> Delay4/1
  Delay2/1 -> HDL Counter1/1, HDL Counter2/1
  Delay1/1 -> HDL Counter1/2, HDL Counter2/2
  Delay3/1 -> HDL Counter2/3
  Delay4/1 -> Logical Operator/1
  Delay9/1 -> HDL Counter1/4, Logical Operator/2
  Delay6/1 -> rx_addr_out/1
  Delay7/1 -> re/1
  HDL Counter1/1 -> Delay8/1
  Delay8/1 -> gs_addr_out/1
  est_step/1 -> Delay9/1
  Constant/1 -> HDL Counter1/3
  gs_sel/1 -> Delay5/1
  Delay5/1 -> gs_sel2/1, gs_sel1/1
  gs_sel1/1 -> select_inputs/1(en1)
  gs_sel2/1 -> select_inputs/2(en2)
  addr1/1 -> Delay10/1
  addr2/1 -> Delay11/1
  Delay10/1 -> select_inputs/3(in1)
  Delay11/1 -> select_inputs/4(in2)
  pd_init/1 -> Delay12/1
  Delay12/1 -> Logical Operator/3

== system ZynqBF_2tx_fpga/channel_estimator/rx_bram ==
  din_i : Inport  OutDataTypeStr=fixdt(1,16,15)
  din_q : Inport  Port=2  OutDataTypeStr=fixdt(1,16,15)
  we : Inport  Port=3  OutDataTypeStr=boolean
  re : Inport  Port=4  OutDataTypeStr=boolean
  rd_addr : Inport  Port=5
  rst : Inport  Port=6  OutDataTypeStr=boolean
  Delay{1..4,6..7} (6 alike) : Delay  DelayLength=1
  Delay5 : Delay  DelayLength=4
  Delay8 : Delay  DelayLength=4
  HDL Counter : hdlsllib/Sources/HDL Counter  CountType=Count limited  CountInit=1  CountStep=1  CountMax=32767  CountFromType=Initial value  CountFrom=1  CountResetPort=on  CountLoadPort=off  CountEnbPort=on  CountDirPort=off  CountDataType=Unsigned  CountWordLen=15  CountFracLen=0  CountSampTime=1
      settings: SourceProductBaseCode=HD
  Vector Concatenate : Concatenate
  rx_ram_i : hdlsllib/HDL RAMs/Simple Dual Port RAM  ram_size=15
      settings: SourceProductName=HDL Coder  SourceProductBaseCode=HD
  rx_ram_q : hdlsllib/HDL RAMs/Simple Dual Port RAM  ram_size=15
      settings: SourceProductName=HDL Coder  SourceProductBaseCode=HD
  dout : Outport
  valid : Outport  Port=2
  addr_out : Outport  Port=3
  wires:
  we/1 -> Delay1/1
  din_q/1 -> Delay4/1
  rx_ram_q/1 -> Delay7/1
  din_i/1 -> Delay3/1
  rd_addr/1 -> Delay8/1, Delay2/1
  rx_ram_i/1 -> Delay6/1
  HDL Counter/1 -> rx_ram_q/2, rx_ram_i/2
  Delay1/1 -> HDL Counter/2, rx_ram_q/3, rx_ram_i/3
  Delay2/1 -> rx_ram_q/4, rx_ram_i/4
  Delay3/1 -> rx_ram_i/1
  Delay4/1 -> rx_ram_q/1
  re/1 -> Delay5/1
  Delay5/1 -> valid/1
  rst/1 -> HDL Counter/1
  Delay7/1 -> Vector Concatenate/2
  Delay8/1 -> addr_out/1
  Vector Concatenate/1 -> dout/1
  Delay6/1 -> Vector Concatenate/1

== system ZynqBF_2tx_fpga/channel_estimator/state_machine ==
  peak_found : Inport
  est_done : Inport  Port=2
  cf_done : Inport  Port=3
  Compare To Constant : simulink/Logic and Bit Operations/Compare To Constant  relop===  const=0  OutDataTypeStr=boolean
  Compare To Constant1 : simulink/Logic and Bit Operations/Compare To Constant  relop===  const=1  OutDataTypeStr=boolean
  Compare To Constant2 : simulink/Logic and Bit Operations/Compare To Constant  relop===  const=2  OutDataTypeStr=boolean
  Delay : Delay  DelayLength=3
  Delay1 : Delay  DelayLength=3
  HDL Counter : hdlsllib/Sources/HDL Counter  CountType=Count limited  CountInit=0  CountStep=1  CountMax=2  CountFromType=Initial value  CountFrom=0  CountResetPort=off  CountLoadPort=off  CountEnbPort=on  CountDirPort=off  CountDataType=Unsigned  CountWordLen=8  CountFracLen=0  CountSampTime=1
      settings: SourceProductBaseCode=HD
  Logical Operator1 : Logic  IconShape=distinctive  AllPortsSameDT=off  OutDataTypeStr=boolean
  Logical Operator3 : Logic  Operator=OR  Inputs=3  IconShape=distinctive  AllPortsSameDT=off  OutDataTypeStr=boolean
  pd_en : Outport
  est_en : Outport  Port=2
  cf_en : Outport  Port=3
  probe_state : Outport  Port=4
  wires:
  est_done/1 -> Delay1/1
  HDL Counter/1 -> probe_state/1, Compare To Constant2/1, Compare To Constant1/1, Compare To Constant/1
  peak_found/1 -> Delay/1
  Logical Operator3/1 -> HDL Counter/1
  Delay/1 -> Logical Operator3/1
  Delay1/1 -> Logical Operator3/2
  Compare To Constant/1 -> pd_en/1
  Compare To Constant1/1 -> est_en/1
  Compare To Constant2/1 -> Logical Operator1/2, cf_en/1
  cf_done/1 -> Logical Operator1/1
  Logical Operator1/1 -> Logical Operator3/3

== system ZynqBF_2tx_fpga/channel_estimator/ch_est/calc_inverse ==
  din : Inport
  en : Inport  Port=2
  Compare To Constant : simulink/Logic and Bit Operations/Compare To Constant  relop===  const=4  OutDataTypeStr=boolean
  Delay18 : Delay  DelayLength=1
  Delay20 : Delay  DelayLength=1
  Delay4 : Delay  DelayLength=1
  HDL Counter : hdlsllib/Sources/HDL Counter  CountType=Count limited  CountInit=0  CountStep=1  CountMax=9  CountFromType=Initial value  CountFrom=0  CountResetPort=on  CountLoadPort=off  CountEnbPort=on  CountDirPort=off  CountDataType=Unsigned  CountWordLen=8  CountFracLen=0  CountSampTime=1
      settings: SourceProductBaseCode=HD
  HDL Reciprocal : Reciprocal  NumberOfIterations=5
  Logical Operator2 : Logic  Operator=NOT  IconShape=distinctive  AllPortsSameDT=off  OutDataTypeStr=boolean
  Switch1 : Switch  Criteria=u2 ~= 0
  dout : Outport
  dval : Outport  Port=2
  wires:
  Logical Operator2/1 -> HDL Counter/1
  Compare To Constant/1 -> Switch1/2, Delay18/1
  HDL Reciprocal/1 -> Switch1/1
  en/1 -> Logical Operator2/1, HDL Counter/2
  HDL Counter/1 -> Compare To Constant/1
  Delay18/1 -> dval/1
  Delay20/1 -> dout/1
  din/1 -> HDL Reciprocal/1
  Switch1/1 -> Delay20/1, Delay4/1
  Delay4/1 -> Switch1/3

== system ZynqBF_2tx_fpga/channel_estimator/ch_est/local_fsm ==
  nr_done : Inport
  dp_done : Inport  Port=2
  Compare To Constant : simulink/Logic and Bit Operations/Compare To Constant  relop===  const=0  OutDataTypeStr=boolean
  Compare To Constant1 : simulink/Logic and Bit Operations/Compare To Constant  relop===  const=1  OutDataTypeStr=boolean
  Compare To Constant2 : simulink/Logic and Bit Operations/Compare To Constant  relop===  const=2  OutDataTypeStr=boolean
  HDL Counter : hdlsllib/Sources/HDL Counter  CountType=Count limited  CountInit=0  CountStep=1  CountMax=2  CountFromType=Initial value  CountFrom=0  CountResetPort=off  CountLoadPort=off  CountEnbPort=on  CountDirPort=off  CountDataType=Unsigned  CountWordLen=8  CountFracLen=0  CountSampTime=1
      settings: SourceProductBaseCode=HD
  Logical Operator : Logic  Operator=OR  Inputs=3  IconShape=distinctive  AllPortsSameDT=off  OutDataTypeStr=boolean
  en_dp : Outport
  en_nr : Outport  Port=2
  en_est : Outport  Port=3
  wires:
  Logical Operator/1 -> HDL Counter/1
  dp_done/1 -> Logical Operator/1
  nr_done/1 -> Logical Operator/2
  HDL Counter/1 -> Compare To Constant/1, Compare To Constant2/1, Compare To Constant1/1
  Compare To Constant/1 -> en_dp/1
  Compare To Constant1/1 -> en_nr/1
  Compare To Constant2/1 -> Logical Operator/3, en_est/1

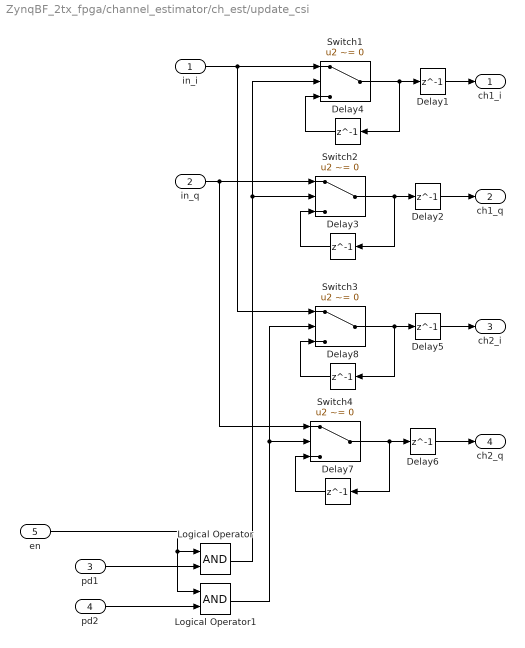
== system ZynqBF_2tx_fpga/channel_estimator/ch_est/update_csi ==
  in_i : Inport
  in_q : Inport  Port=2
  pd1 : Inport  Port=3
  pd2 : Inport  Port=4
  en : Inport  Port=5
  Delay{1..8} (8 alike) : Delay  DelayLength=1
  Logical Operator : Logic  AllPortsSameDT=off  OutDataTypeStr=boolean
  Logical Operator1 : Logic  AllPortsSameDT=off  OutDataTypeStr=boolean
  Switch{1..4} (4 alike) : Switch  Criteria=u2 ~= 0
  ch1_i : Outport
  ch1_q : Outport  Port=2
  ch2_i : Outport  Port=3
  ch2_q : Outport  Port=4
  wires:
  pd1/1 -> Logical Operator/2
  en/1 -> Logical Operator1/1, Logical Operator/1
  Logical Operator/1 -> Switch1/2, Switch2/2
  pd2/1 -> Logical Operator1/2
  Switch1/1 -> Delay1/1, Delay4/1
  Delay4/1 -> Switch1/3
  Delay1/1 -> ch1_i/1
  Delay2/1 -> ch1_q/1
  Switch2/1 -> Delay2/1, Delay3/1
  Delay3/1 -> Switch2/3
  Switch3/1 -> Delay5/1, Delay8/1
  in_i/1 -> Switch3/1, Switch1/1
  in_q/1 -> Switch4/1, Switch2/1
  Delay7/1 -> Switch4/3
  Delay8/1 -> Switch3/3
  Delay5/1 -> ch2_i/1
  Switch4/1 -> Delay6/1, Delay7/1
  Delay6/1 -> ch2_q/1
  Logical Operator1/1 -> Switch3/2, Switch4/2

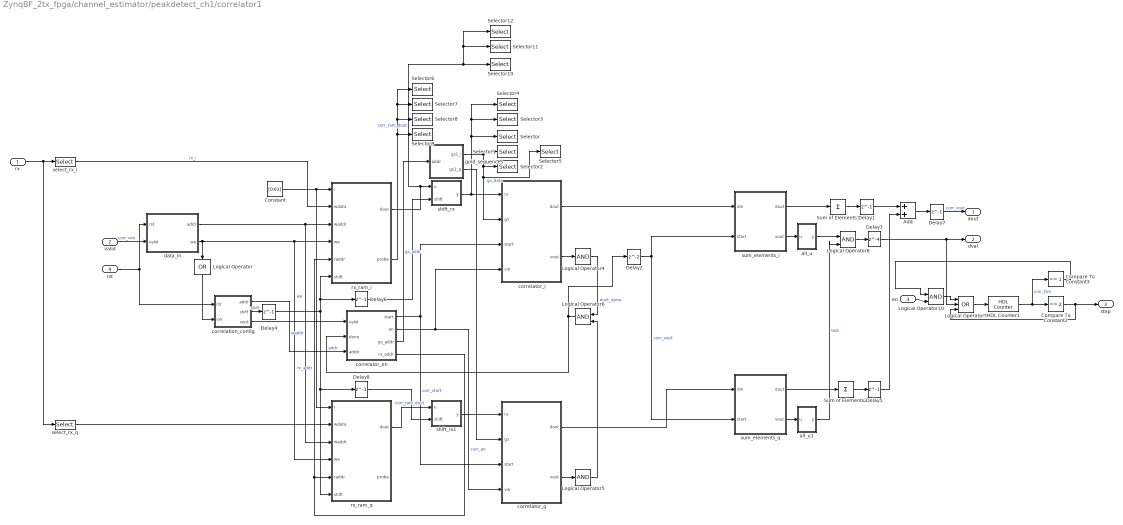
== system ZynqBF_2tx_fpga/channel_estimator/peakdetect_ch1/correlator1 ==
  rx : Inport
  valid : Inport  Port=2
  en : Inport  Port=3
  rst : Inport  Port=4
  Add : Sum  OutDataTypeStr=fixdt(1,32,16)
  Compare To Constant2 : simulink/Logic and Bit Operations/Compare To Constant  relop===  const=2  OutDataTypeStr=boolean
  Compare To Constant3 : simulink/Logic and Bit Operations/Compare To Constant  relop===  const=1  OutDataTypeStr=boolean
  Constant : Constant  Value=[0:63]  OutDataTypeStr=fixdt(0,6,0)  SampleTime=-1
  Delay{1,4..8} (6 alike) : Delay  DelayLength=1
  Delay2 : Delay
  Delay3 : Delay  DelayLength=4
  HDL Counter1 : hdlsllib/Sources/HDL Counter  CountType=Count limited  CountInit=0  CountStep=1  CountMax=2  CountFromType=Initial value  CountFrom=0  CountResetPort=off  CountLoadPort=off  CountEnbPort=on  CountDirPort=off  CountDataType=Unsigned  CountWordLen=8  CountFracLen=0  CountSampTime=1
      settings: SourceProductBaseCode=HD
  Logical Operator : Logic  Operator=OR  Inputs=1  IconShape=distinctive  AllPortsSameDT=off  OutDataTypeStr=boolean
  Logical Operator10 : Logic  IconShape=distinctive  AllPortsSameDT=off  OutDataTypeStr=boolean
  Logical Operator4 : Logic  Inputs=1  IconShape=distinctive  AllPortsSameDT=off  OutDataTypeStr=boolean
  Logical Operator5 : Logic  Inputs=1  IconShape=distinctive  AllPortsSameDT=off  OutDataTypeStr=boolean
  Logical Operator6 : Logic  IconShape=distinctive  AllPortsSameDT=off  OutDataTypeStr=boolean
  Logical Operator8 : Logic  IconShape=distinctive  AllPortsSameDT=off  OutDataTypeStr=boolean
  Logical Operator9 : Logic  Operator=OR  Inputs=3  IconShape=distinctive  AllPortsSameDT=off  OutDataTypeStr=boolean
  Selector{,1,9..10} (4 alike) : Selector  IndexMode=Zero-based  InputPortWidth=64  IndexOptions=Starting index (dialog)  Indices=[63]  OutputSizes=1
  Selector{2..3,6,11} (4 alike) : Selector  IndexMode=Zero-based  InputPortWidth=64  IndexOptions=Starting index (dialog)  Indices=[0]  OutputSizes=1
  Selector{4..5,8,12} (4 alike) : Selector  IndexMode=Zero-based  InputPortWidth=64  IndexOptions=Starting index (dialog)  Indices=[62]  OutputSizes=1
  Selector7 : Selector  IndexMode=Zero-based  InputPortWidth=64  IndexOptions=Starting index (dialog)  Indices=[1]  OutputSizes=1
  Sum of Elements1 : Sum  Inputs=+
  Sum of Elements2 : Sum  Inputs=+
  all_u : MATLAB Function  TreatAsAtomicUnit=on
  all_u1 : MATLAB Function  TreatAsAtomicUnit=on
  correlation_config : Subsystem
  correlator_en : Subsystem
  correlator_i : Subsystem  TreatAsAtomicUnit=on
  correlator_q : Subsystem  TreatAsAtomicUnit=on
  data_in : Subsystem
  gold_sequences : Subsystem
  rx_ram_i : Subsystem  TreatAsAtomicUnit=on
  rx_ram_q : Subsystem  TreatAsAtomicUnit=on
  select_rx_i : Selector  IndexMode=Zero-based  InputPortWidth=2  IndexOptions=Index vector (dialog)  Indices=[0]  OutputSizes=1
  select_rx_q : Selector  IndexMode=Zero-based  InputPortWidth=2  IndexOptions=Index vector (dialog)  Indices=[1]  OutputSizes=1
  shift_rx : MATLAB Function  TreatAsAtomicUnit=on
  shift_rx1 : MATLAB Function  TreatAsAtomicUnit=on
  sum_elements_i : Subsystem  TreatAsAtomicUnit=on
  sum_elements_q : Subsystem  TreatAsAtomicUnit=on
  dout : Outport
  dval : Outport  Port=2
  step : Outport  Port=3
  wires:
  rx_ram_i/1(dout) -> shift_rx/1(u), Selector10/1, Selector11/1, Selector12/1  "corr_ram_dout"
  rx/1 -> select_rx_q/1, select_rx_i/1
  select_rx_i/1 -> rx_ram_i/2(wdata)  "rx_i"
  data_in/1(addr) -> rx_ram_q/3(waddr), rx_ram_i/3(waddr)  "waddr"
  data_in/2(we) -> rx_ram_q/4(we), rx_ram_i/4(we), Logical Operator/1  "we"
  rst/1 -> correlation_config/1(rst), data_in/1(rst)
  Constant/1 -> rx_ram_q/1(i), rx_ram_i/1(i)
  valid/1 -> data_in/2(valid)  "corr_vim"
  Logical Operator/1 -> correlation_config/2(vin)
  correlator_en/1(start) -> correlator_q/3(start), correlator_i/3(start)  "corr_start"
  correlator_en/2(en) -> correlator_q/4(vin), correlator_i/4(vin)  "corr_en"
  correlation_config/2(shift) -> Delay4/1  "shift"
  correlation_config/3(vout) -> correlator_en/1(valid)
  correlation_config/1(addr) -> correlator_en/3(addri)  "addr"
  correlator_en/4(rx_addr) -> rx_ram_i/5(raddr), rx_ram_q/5(raddr)  "rx_addr"
  correlator_en/3(gs_addr) -> gold_sequences/1(addr)  "gs_addr"
  gold_sequences/1(gs1_i) -> Selector5/1, correlator_i/2(gs), Selector2/1, Selector1/1  "gs_data"
  correlator_i/1(dout) -> sum_elements_i/1(din)
  Delay2/1 -> sum_elements_i/2(start), sum_elements_q/2(start)  "corr_vout"
  rx_ram_i/2(probe) -> Selector9/1, Selector8/1, Selector7/1, Selector6/1
  shift_rx/1(y) -> Selector/1, Selector3/1, Selector4/1, correlator_i/1(rx)
  correlator_i/2(vout) -> Logical Operator4/1
  Sum of Elements1/1 -> Delay1/1
  Delay1/1 -> Add/1
  select_rx_q/1 -> rx_ram_q/2(wdata)
  rx_ram_q/1(dout) -> shift_rx1/1(u)  "corr_ram_dout"
  shift_rx1/1(y) -> correlator_q/1(rx)
  gold_sequences/2(gs1_q) -> correlator_q/2(gs)
  correlator_q/2(vout) -> Logical Operator5/1
  Logical Operator4/1 -> Logical Operator6/1  "mult_done"
  Logical Operator5/1 -> Logical Operator6/2
  Logical Operator6/1 -> correlator_en/2(done), Delay2/1
  Delay5/1 -> Add/2
  Sum of Elements2/1 -> Delay5/1
  correlator_q/1(dout) -> sum_elements_q/1(din)
  Add/1 -> Delay7/1
  Delay7/1 -> dout/1  "corr_vout"
  sum_elements_i/2(vout) -> all_u/1(u)
  sum_elements_i/1(dout) -> Sum of Elements1/1
  sum_elements_q/1(dout) -> Sum of Elements2/1
  sum_elements_q/2(vout) -> all_u1/1(u)
  all_u/1(y) -> Logical Operator8/1
  Logical Operator8/1 -> Delay3/1
  all_u1/1(y) -> Logical Operator8/2  "test"
  Delay3/1 -> Logical Operator9/2, dval/1
  HDL Counter1/1 -> Compare To Constant3/1, Compare To Constant2/1  "corr_fsm"
  Compare To Constant2/1 -> Logical Operator9/3, step/1
  Logical Operator9/1 -> HDL Counter1/1
  en/1 -> Logical Operator10/2
  Logical Operator10/1 -> Logical Operator9/1
  Compare To Constant3/1 -> Logical Operator10/1
  Delay4/1 -> Delay6/1, rx_ram_i/6(shift), Delay8/1, rx_ram_q/6(shift)
  Delay6/1 -> shift_rx/2(shift)
  Delay8/1 -> shift_rx1/2(shift)

== system ZynqBF_2tx_fpga/channel_estimator/peakdetect_ch1/peak_fsm ==
  t_cross : Inport
  cnt_end : Inport  Port=2
  Compare To Constant : simulink/Logic and Bit Operations/Compare To Constant  relop===  const=1  OutDataTypeStr=boolean
  Compare To Constant1 : simulink/Logic and Bit Operations/Compare To Constant  relop===  const=0  OutDataTypeStr=boolean
  Compare To Constant2 : simulink/Logic and Bit Operations/Compare To Constant  relop===  const=2  OutDataTypeStr=boolean
  HDL Counter : hdlsllib/Sources/HDL Counter  CountType=Count limited  CountInit=0  CountStep=1  CountMax=3  CountFromType=Initial value  CountFrom=0  CountResetPort=off  CountLoadPort=off  CountEnbPort=on  CountDirPort=off  CountDataType=Unsigned  CountWordLen=8  CountFracLen=0  CountSampTime=1
      settings: SourceProductBaseCode=HD
  Logical Operator : Logic  IconShape=distinctive  AllPortsSameDT=off  OutDataTypeStr=boolean
  Logical Operator1 : Logic  Operator=OR  Inputs=3  IconShape=distinctive  AllPortsSameDT=off  OutDataTypeStr=boolean
  scan_peak : Outport
  peak_found : Outport  Port=2
  wires:
  HDL Counter/1 -> Compare To Constant2/1, Compare To Constant/1, Compare To Constant1/1
  Compare To Constant1/1 -> Logical Operator/2
  t_cross/1 -> Logical Operator/1
  Compare To Constant/1 -> scan_peak/1
  Logical Operator1/1 -> HDL Counter/1
  Logical Operator/1 -> Logical Operator1/3
  cnt_end/1 -> Logical Operator1/2
  Compare To Constant2/1 -> Logical Operator1/1, peak_found/1

== system ZynqBF_2tx_fpga/channel_estimator/peakdetect_ch1/running_max ==
  din : Inport
  en : Inport  Port=2
  rst : Inport  Port=3
  Constant : Constant  Value=0  OutDataTypeStr=fixdt(1,32,16)  SampleTime=-1
  Delay4 : Delay  DelayLength=1
  Relational Operator : RelationalOperator  Operator=>  OutDataTypeStr=boolean  RndMeth=Nearest
  reset_max : Switch  Criteria=u2 ~= 0
  store_max : Switch  Criteria=u2 ~= 0
  update_max : Logic  IconShape=distinctive  AllPortsSameDT=off  OutDataTypeStr=boolean
  new_max : Outport
  max_val : Outport  Port=2
  wires:
  reset_max/1 -> Delay4/1
  Constant/1 -> reset_max/1
  Relational Operator/1 -> update_max/2
  store_max/1 -> reset_max/3
  Delay4/1 -> store_max/3, max_val/1, Relational Operator/2
  en/1 -> update_max/1
  din/1 -> store_max/1, Relational Operator/1
  rst/1 -> reset_max/2
  update_max/1 -> new_max/1, store_max/2  "update_max_p"

== system ZynqBF_2tx_fpga/channel_estimator/peakdetect_ch1/store_index ==
  din : Inport
  update : Inport  Port=2
  Delay{1..2,4..5} (4 alike) : Delay  DelayLength=1
  Switch : Switch  Criteria=u2 ~= 0
  dout : Outport
  wires:
  Delay5/1 -> Switch/3
  update/1 -> Delay1/1
  din/1 -> Delay2/1
  Switch/1 -> Delay4/1, Delay5/1
  Delay2/1 -> Switch/1
  Delay1/1 -> Switch/2
  Delay4/1 -> dout/1
